simulink model "blockdemo"  (Simulink 6.3)
settings: Solver=FixedStepDiscrete  StartTime=0  StopTime=1200  FixedStep=1  RelTol=1e-3
InitFcn:
  | %% DSPBuilder Start
  | alt_dspbuilder_update_model(bdroot)
  | %% DSPBuilder End
libraries: allblocks_alteradspbuilder2 x10, simulink x1
settings Model: Creator=mjervis  LastModifiedBy=delphick
settings DebuggingCC: MultiTaskDSMMsg=error

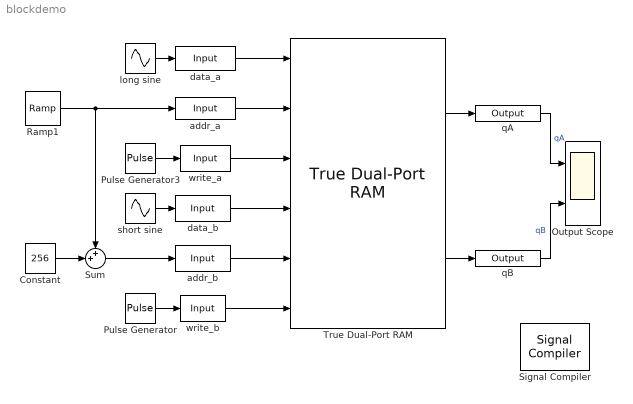
== system blockdemo ==
  Constant : Constant  Value=256
  Output Scope : Scope  NumInputPorts=2
      settings: TimeRange=1200  YMin=-1~-1  YMax=1~1  SampleInput=on  SampleTime=1
  Pulse Generator : DiscretePulseGenerator  Period=512  PulseWidth=256  PhaseDelay=128
  Pulse Generator3 : DiscretePulseGenerator  Period=512  PulseWidth=256
  Ramp1 : simulink/Sources/Ramp  slope=0.5  start=0  X0=0
  Signal Compiler : allblocks_alteradspbuilder2/Signal Compiler  DeviceFamily=Stratix III  DeviceName=AUTO  EnableSignalTap=off  SignalTapDepth=128  UseBoardBlock=off  StpUseDefaultClock=on  StpClock=clock
  Sum : Sum  Inputs=++|
  True Dual-Port RAM : allblocks_alteradspbuilder2/True Dual-Port RAM  numwords=512  BusType=Signed Fractional  bwl=2  bwr=30  memory_type=AUTO  ram_type=TrueDualRAM  initialization=Blank  init_file=input.hex  init_array=[7:-1:0]  register_outputs=on  use_ena=off  ClockPhase=1
      settings: AttributesFormatString=Initialization = %<initialization>\nRegister Outputs = %<register_outputs>
  addr_a : allblocks_alteradspbuilder2/Input  iofile=C:\workspace_clean\Documentation\DesignExamples\Tutorials\UnitBlocks\Storage\TrueDualPortRAM\tb_blockdemo\blockdemo_addr_a.salt  BusType=Unsigned Integer  bwl=9  bwr=0  SpecifyClock=off  clock=default_clock  PORTTYPE=Input
  addr_b : allblocks_alteradspbuilder2/Input  iofile=C:\workspace_clean\Documentation\DesignExamples\Tutorials\UnitBlocks\Storage\TrueDualPortRAM\tb_blockdemo\blockdemo_addr_b.salt  BusType=Unsigned Integer  bwl=9  bwr=0  SpecifyClock=off  clock=default_clock  PORTTYPE=Input
  data_a : allblocks_alteradspbuilder2/Input  iofile=C:\workspace_clean\Documentation\DesignExamples\Tutorials\UnitBlocks\Storage\TrueDualPortRAM\tb_blockdemo\blockdemo_data_a.salt  BusType=Signed Fractional  bwl=2  bwr=30  SpecifyClock=off  clock=default_clock  PORTTYPE=Input
  data_b : allblocks_alteradspbuilder2/Input  iofile=C:\workspace_clean\Documentation\DesignExamples\Tutorials\UnitBlocks\Storage\TrueDualPortRAM\tb_blockdemo\blockdemo_data_b.salt  BusType=Signed Fractional  bwl=2  bwr=30  SpecifyClock=off  clock=default_clock  PORTTYPE=Input
  long sine : Sin  SineType=Sample based  Samples=100  SampleTime=1
  qA : allblocks_alteradspbuilder2/Output  iofile=C:\workspace_clean\Documentation\DesignExamples\Tutorials\UnitBlocks\Storage\TrueDualPortRAM\tb_blockdemo\blockdemo_qA.capture  BusType=Inferred  bwl=8  bwr=0  PORTTYPE=Output
  qB : allblocks_alteradspbuilder2/Output  iofile=C:\workspace_clean\Documentation\DesignExamples\Tutorials\UnitBlocks\Storage\TrueDualPortRAM\tb_blockdemo\blockdemo_qB.capture  BusType=Inferred  bwl=8  bwr=0  PORTTYPE=Output
  short sine : Sin  SineType=Sample based  Amplitude=0.5  SampleTime=1
  write_a : allblocks_alteradspbuilder2/Input  iofile=C:\workspace_clean\Documentation\DesignExamples\Tutorials\UnitBlocks\Storage\TrueDualPortRAM\tb_blockdemo\blockdemo_write_a.salt  BusType=Single Bit  bwl=3  bwr=0  SpecifyClock=off  clock=default_clock  PORTTYPE=Input
  write_b : allblocks_alteradspbuilder2/Input  iofile=C:\workspace_clean\Documentation\DesignExamples\Tutorials\UnitBlocks\Storage\TrueDualPortRAM\tb_blockdemo\blockdemo_write_b.salt  BusType=Single Bit  bwl=3  bwr=0  SpecifyClock=off  clock=default_clock  PORTTYPE=Input
  wires:
  data_a/1 -> True Dual-Port RAM/1
  addr_a/1 -> True Dual-Port RAM/2
  addr_b/1 -> True Dual-Port RAM/5
  write_b/1 -> True Dual-Port RAM/6
  Pulse Generator/1 -> write_b/1
  Ramp1/1 -> addr_a/1, Sum/1
  long sine/1 -> data_a/1
  True Dual-Port RAM/1 -> qA/1
  data_b/1 -> True Dual-Port RAM/4
  Pulse Generator3/1 -> write_a/1
  write_a/1 -> True Dual-Port RAM/3
  short sine/1 -> data_b/1
  Sum/1 -> addr_b/1
  True Dual-Port RAM/2 -> qB/1
  qA/1 -> Output Scope/1  "qA"
  qB/1 -> Output Scope/2  "qB"
  Constant/1 -> Sum/2
